simulink model "integ_gain_slew_test"  (Simulink 8.1)
settings: Solver=ode45  StartTime=0.0  StopTime=10.0  RelTol=1e-3
values from neighbouring files (symbols this model uses):
  alfa = Cin/(Co+(Co+Cin)/A)    (= 0.999800039992)    [integ_slew_test.m]
  gamma = 1/(1+Cin/((A+1)*Co))    (= 0.999900019996)    [integ_slew_test.m]
  GBW = 1    [integ_slew_test.m]
  SR = 10    [integ_slew_test.m]
  Ts = 1    [integ_slew_test.m]
  VinHi = 2    [integ_slew_test.m]
undefined symbols (not defined in the file or in its folder): slew
settings Model: Creator=yasuda  LastModifiedBy=anagix
settings OptimizationCC: InitFltsAndDblsToZero=on
settings DebuggingCC: SaveWithParameterizedLinksMsg=none  StrictBusMsg=Warning
settings GRTTargetCC: TargetFcnLib=ansi_tfl_tmw.mat

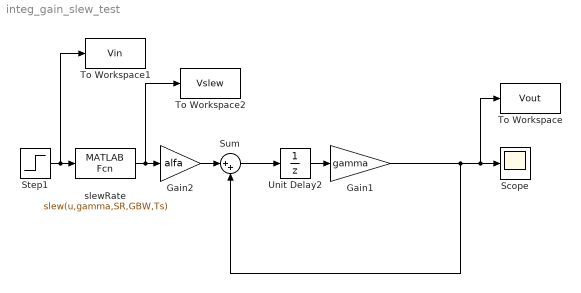
== system integ_gain_slew_test ==
  Gain1 : Gain  Gain=gamma
  Gain2 : Gain  Gain=alfa
  Scope : Scope
  Step1 : Step  After=VinHi  SampleTime=0
  Sum : Sum  Inputs=|++
  To Workspace : ToWorkspace  VariableName=Vout  SampleTime=1
  To Workspace1 : ToWorkspace  VariableName=Vin  SampleTime=1
  To Workspace2 : ToWorkspace  VariableName=Vslew  SampleTime=1
  Unit Delay2 : UnitDelay  SampleTime=Ts
  slewRate : MATLABFcn  MATLABFcn=slew(u,gamma,SR,GBW,Ts)
  wires:
  Sum/1 -> Unit Delay2/1
  Unit Delay2/1 -> Gain1/1
  Gain1/1 -> Sum/2, Scope/1, To Workspace/1
  Gain2/1 -> Sum/1
  slewRate/1 -> Gain2/1, To Workspace2/1
  Step1/1 -> slewRate/1, To Workspace1/1
